simulink model "simFLC"  (R2023b)
settings: Solver=VariableStepAuto  StartTime=0.0  StopTime=7  RelTol=1e-3
undefined symbols (not defined in the file): IntegralGain, ProportionalGain
libraries: slpidlib x1, fuzblock x1
settings Model: Creator=minakosm  LastModifiedBy=yiannislevy
settings OptimizationCC: ReuseModelBlockBuffer=off

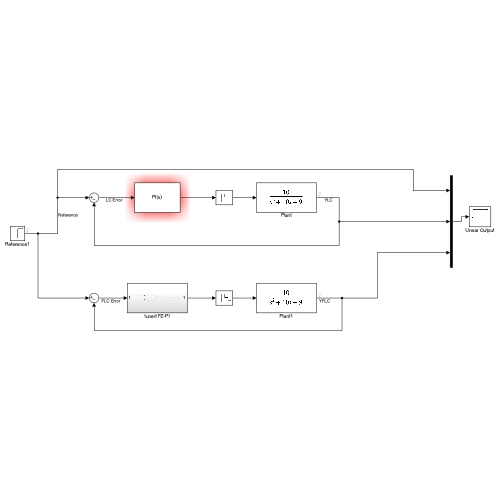
[thumbnail: Simulink's stored preview of the top-level diagram]
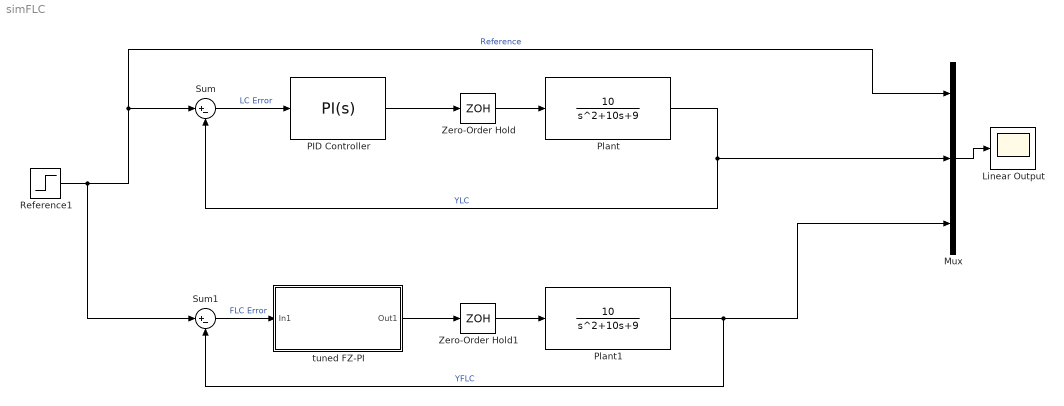
== system simFLC ==
  Linear Output : Scope
  Mux : Mux  Inputs=3
  PID Controller : slpidlib/PID Controller  Controller=PI  Form=Parallel  TimeDomain=Continuous-time  UseExternalTs=off  SampleTime=-1  IntegratorMethod=Forward Euler  FilterMethod=Forward Euler  ControllerParametersSource=internal  P=ProportionalGain  I=IntegralGain  UseKiTs=off  D=0  N=100  UseFilter=on  TunerSelectOption=Transfer Function Based (PID Tuner App)  InitialConditionSource=internal  InitialConditionForIntegrator=0  InitialConditionForFilter=0  DifferentiatorICPrevScaledInput=0  ExternalReset=none  TrackingMode=off  Kt=1  LimitOutput=off  SatLimitsSource=internal  UpperSaturationLimit=inf  LowerSaturationLimit=-inf  LinearizeAsGain=on  AntiWindupMode=none  Kb=1  LimitIntegrator=off  UpperIntegratorSaturationLimit=inf  LowerIntegratorSaturationLimit=-inf  POutMin=[]  POutMax=[]  IOutMin=[]  IOutMax=[]  DOutMin=[]  DOutMax=[]  NOutMin=[]  NOutMax=[]  SumOutMin=[]  SumOutMax=[]  SaturationOutMin=[]  SaturationOutMax=[]  PParamMin=[]  PParamMax=[]  IParamMin=[]  IParamMax=[]  DParamMin=[]  DParamMax=[]  NParamMin=[]  NParamMax=[]  KbParamMin=[]  KbParamMax=[]  KtParamMin=[]  KtParamMax=[]  KbOutMin=[]  KbOutMax=[]  KtOutMin=[]  KtOutMax=[]  IntegratorOutMin=[]  IntegratorOutMax=[]  FilterOutMin=[]  FilterOutMax=[]  SumI1OutMin=[]  SumI1OutMax=[]  SumI2OutMin=[]  SumI2OutMax=[]  SumI3OutMin=[]  SumI3OutMax=[]  SumI4OutMin=[]  SumI4OutMax=[]  SumDOutMin=[]  SumDOutMax=[]  DifferentiatorOutMin=[]  DifferentiatorOutMax=[]  FilterDiffOutCoefMin=[]  FilterDiffOutCoefMax=[]  ReciprocalOutMin=[]  ReciprocalOutMax=[]  SumDenOutMin=[]  SumDenOutMax=[]  SumNumOutMin=[]  SumNumOutMax=[]  DivideOutMin=[]  DivideOutMax=[]  UdiffTsProdOutMin=[]  UdiffTsProdOutMax=[]  NTsProdOutMin=[]  NTsProdOutMax=[]  UintegralTsProdOutMin=[]  UintegralTsProdOutMax=[]  UngainTsProdOutMin=[]  UngainTsProdOutMax=[]  ClampingZeroOutDataTypeStr=Inherit: Inherit via back propagation  ClampingZeroOutMin=[]  ClampingZeroOutMax=[]  FilterDenConstantOutDataTypeStr=Inherit: Inherit via back propagation  FilterDenConstantOutMin=[]  FilterDenConstantOutMax=[]  PCopyOutDataTypeStr=Inherit: Inherit via back propagation  PCopyOutMin=[]  PCopyOutMax=[]  NCopyOutDataTypeStr=Inherit: Inherit via back propagation  NCopyOutMin=[]  NCopyOutMax=[]  IntegratorContinuousStateAttributes=''  IntegratorStateMustResolveToSignalObject=off  IntegratorRTWStateStorageClass=Auto  FilterContinuousStateAttributes=''  FilterStateMustResolveToSignalObject=off  FilterRTWStateStorageClass=Auto  ParallelPVariant=InternalParameters  IdealPVariant=Disabled  IVariant=InternalParameters  DVariant=Disabled  IntegratorVariant=Continuous  SatVariant=Disabled  AWVariant=Passthrough  PCopyVariant=Disabled  TRVariant=Disabled  FdbkBlocksVariant=Forward  IdealPFdbkVariant=Disabled  SatFdbkVariant=Disabled  DerivativeFilterVariant=Disabled  NVariant=Disabled  NCopyVariant=Disabled_SignalSpec  FilterICVariant=Disabled  IntegratorICVariant=InternalICs  ExternalResetVariant=Disabled  TRSumVariant=Passthrough  SumFdbkVariant=Disabled  SumVariant=Sum_PI  TsampFilterVariant=InternalTs  TsampNgainVariant=Passthrough  TsampIntegralVariant=Disabled_SignalSpec  ExternalSaturationOutDataTypeStr=Inherit: Same as second input
  Plant : TransferFcn  Numerator=[10]  Denominator=[1 10 9]
  Plant1 : TransferFcn  Numerator=[10]  Denominator=[1 10 9]
  Reference1 : Step  Time=0.1  SampleTime=0.01
  Sum : Sum  Inputs=|+-
  Sum1 : Sum  Inputs=|+-
  Zero-Order Hold : ZeroOrderHold  SampleTime=-1
  Zero-Order Hold1 : ZeroOrderHold  SampleTime=-1
  tuned FZ-PI : Subsystem
  wires:
  Sum1/1 -> tuned FZ-PI/1(In1)  "FLC Error"
  tuned FZ-PI/1(Out1) -> Zero-Order Hold1/1
  Zero-Order Hold1/1 -> Plant1/1
  Plant1/1 -> Mux/3, Sum1/2  "YFLC"
  Mux/1 -> Linear Output/1
  PID Controller/1 -> Zero-Order Hold/1
  Plant/1 -> Sum/2, Mux/2  "YLC"
  Zero-Order Hold/1 -> Plant/1
  Sum/1 -> PID Controller/1  "LC Error"
  Reference1/1 -> Sum1/1, Mux/1, Sum/1  "Reference"

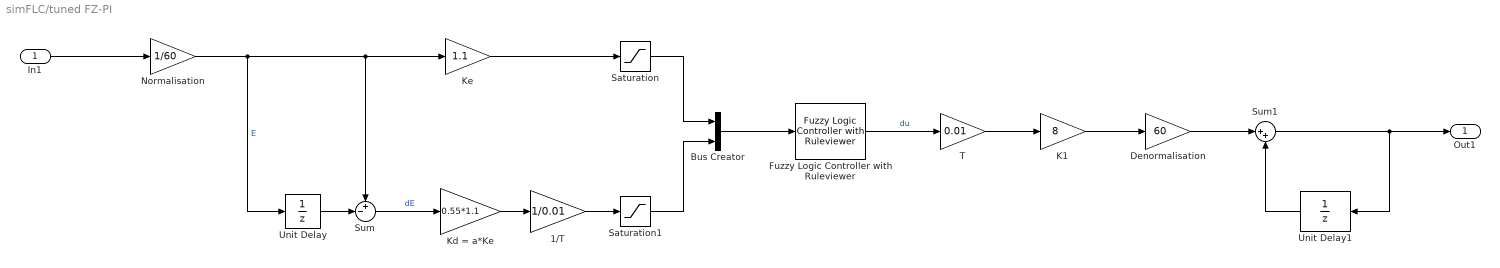
== system simFLC/tuned FZ-PI ==
  In1 : Inport
  1/T : Gain  Gain=1/0.01
  Bus Creator : BusCreator  Inputs=2
  Denormalisation : Gain  Gain=60
  Fuzzy Logic Controller with Ruleviewer : fuzblock/Fuzzy Logic  Controller  with Ruleviewer  fismatrix=FLC  Ts=0.01
  K1 : Gain  Gain=8
  Kd = a*Ke : Gain  Gain=0.55*1.1
  Ke : Gain  Gain=1.1
  Normalisation : Gain  Gain=1/60
  Saturation : Saturate  UpperLimit=1  LowerLimit=-1
  Saturation1 : Saturate  UpperLimit=1  LowerLimit=-1
  Sum : Sum  Inputs=+-|
  Sum1 : Sum  Inputs=|++
  T : Gain  Gain=0.01
  Unit Delay : UnitDelay  SampleTime=-1  HasFrameUpgradeWarning=on
  Unit Delay1 : UnitDelay  SampleTime=-1  HasFrameUpgradeWarning=on
  Out1 : Outport
  wires:
  In1/1 -> Normalisation/1
  K1/1 -> Denormalisation/1
  Unit Delay/1 -> Sum/2
  Saturation1/1 -> Bus Creator/2
  Sum1/1 -> Out1/1, Unit Delay1/1
  T/1 -> K1/1
  Bus Creator/1 -> Fuzzy Logic Controller with Ruleviewer/1
  1/T/1 -> Saturation1/1
  Fuzzy Logic Controller with Ruleviewer/1 -> T/1  "du"
  Saturation/1 -> Bus Creator/1
  Sum/1 -> Kd = a*Ke/1  "dE"
  Normalisation/1 -> Ke/1, Sum/1, Unit Delay/1  "E"
  Ke/1 -> Saturation/1
  Unit Delay1/1 -> Sum1/2
  Denormalisation/1 -> Sum1/1
  Kd = a*Ke/1 -> 1/T/1
